simulink model "Sim_exercise3"  (R2016a)
settings: Solver=VariableStepAuto  StartTime=0.0  StopTime=0.1  RelTol=1e-3
undefined symbols (not defined in the file): dm, Jeq, Kemf, Km, n, R, Tc, voltage
settings Model: Creator=sofianh  LastModifiedBy=Sofía
settings DataIOCC: LimitDataPoints=on
settings DebuggingCC: AllowSymbolicDim=off
settings ModelReferenceCC: PropagateSignalLabelsOutOfModel=off
settings GRTTargetCC: GeneratePreprocessorConditionals=Use local settings

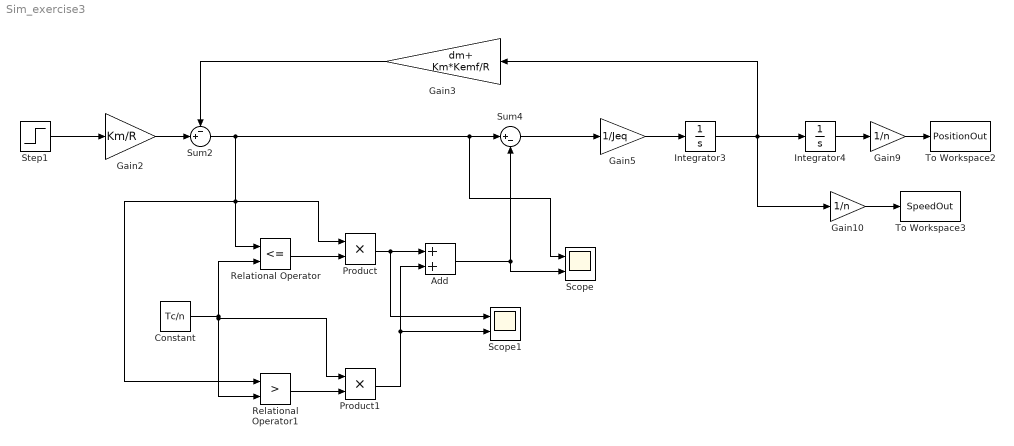
== system Sim_exercise3 ==
  Add : Sum
  Constant : Constant  Value=Tc/n
  Gain10 : Gain  Gain=1/n
  Gain2 : Gain  Gain=Km/R
  Gain3 : Gain  Gain=dm+ Km*Kemf/R
  Gain5 : Gain  Gain=1/Jeq
  Gain9 : Gain  Gain=1/n
  Integrator3 : Integrator
  Integrator4 : Integrator
  Product : Product
  Product1 : Product
  Relational Operator : RelationalOperator  Operator=<=  OutDataTypeStr=boolean
  Relational Operator1 : RelationalOperator  Operator=>  OutDataTypeStr=boolean
  Scope : Scope  NumInputPorts=2
  Scope1 : Scope  NumInputPorts=2
  Step1 : Step  Time=0  After=voltage  SampleTime=0
  Sum2 : Sum  Inputs=-+|
  Sum4 : Sum  Inputs=|+-
  To Workspace2 : ToWorkspace  VariableName=PositionOut  SaveFormat=Structure With Time  SampleTime=-1
  To Workspace3 : ToWorkspace  VariableName=SpeedOut  SaveFormat=Structure With Time  SampleTime=-1
  wires:
  Gain2/1 -> Sum2/2
  Integrator3/1 -> Integrator4/1, Gain10/1, Gain3/1
  Gain3/1 -> Sum2/1
  Relational Operator/1 -> Product/2
  Sum4/1 -> Gain5/1
  Gain5/1 -> Integrator3/1
  Integrator4/1 -> Gain9/1
  Gain9/1 -> To Workspace2/1
  Gain10/1 -> To Workspace3/1
  Step1/1 -> Gain2/1
  Add/1 -> Sum4/2, Scope/2
  Sum2/1 -> Scope/1, Sum4/1, Relational Operator/1, Relational Operator1/1, Product/1
  Constant/1 -> Relational Operator/2, Relational Operator1/2, Product1/1
  Relational Operator1/1 -> Product1/2
  Product/1 -> Scope1/1, Add/1
  Product1/1 -> Scope1/2, Add/2
